simulink model "MioProgettoNew"  (R2023a)
settings: Solver=VariableStepAuto  StartTime=0.0  StopTime=10.0  RelTol=1e-3
settings Model: Creator=bened  LastModifiedBy=bened

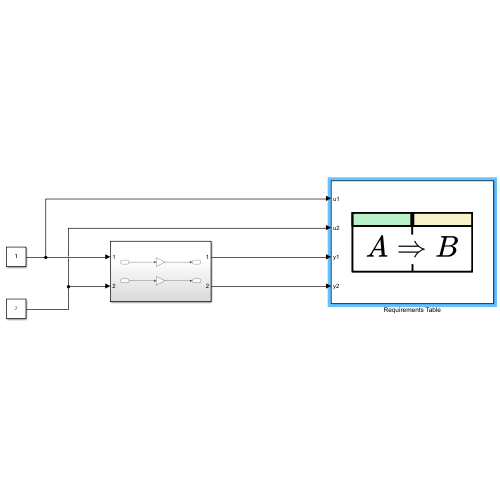
[thumbnail: Simulink's stored preview of the top-level diagram]
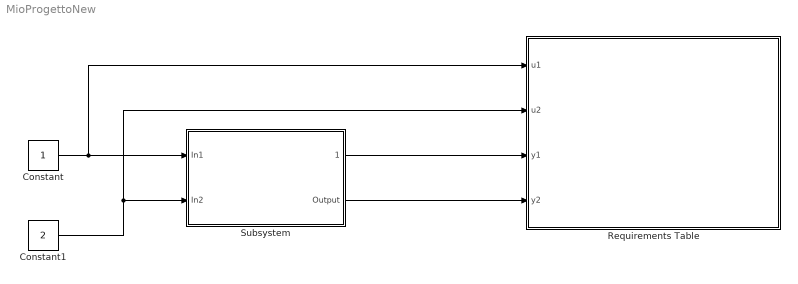
== system MioProgettoNew ==
  Constant : Constant
  Constant1 : Constant  Value=2
  Requirements Table : Requirements Table  TreatAsAtomicUnit=on
  Subsystem : Subsystem
  wires:
  Subsystem/2(Output) -> Requirements Table/4(y2)
  Subsystem/1(1) -> Requirements Table/3(y1)
  Constant/1 -> Requirements Table/1(u1), Subsystem/1(In1)
  Constant1/1 -> Subsystem/2(In2), Requirements Table/2(u2)

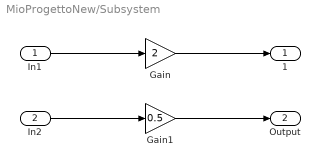
== system MioProgettoNew/Subsystem ==
  In1 : Inport
  In2 : Inport  Port=2
  Gain : Gain  Gain=2
  Gain1 : Gain  Gain=0.5
  1 : Outport
  Output : Outport  Port=2
  wires:
  In1/1 -> Gain/1
  Gain/1 -> 1/1
  In2/1 -> Gain1/1
  Gain1/1 -> Output/1

== stateflow chart MioProgettoNew/Requirements Table ==
  (default) -> (junction 1073741860)
  (junction 1073741860) -> (junction 1073741861) : {
      | % SF_REQ_REV_07
      | }
  (junction 1073741861) -> (junction 1073741863) : {
      | % HEADER_ASSIGNMENTS
      |
      | }
  (junction 1073741863) -> (junction 1073741865) : {
      | % START_A_4
      | }
  (junction 1073741865) -> (junction 1073741867) : {
      | }
  (junction 1073741867) -> (junction 1073741869)
  (junction 1073741869) -> (junction 1073741871) : {
      | }
  (junction 1073741871) -> (junction 1073741873) : {
      | % END_A_4
      | }
  (junction 1073741873) -> (junction 1073741919) : {
      | % START_R_1
      | }
  (junction 1073741919) -> (junction 1073741921) : {
      | }
  (junction 1073741921) -> (junction 1073741923)
  (junction 1073741923) -> (junction 1073741925) [order 1] : [(u1 > 0)]
  (junction 1073741923) -> (junction 1073741931) [order 2]
  (junction 1073741925) -> (junction 1073741927) : {
      | reqtable_postcondition((y1 > 0), 'R:1');
      |
      |
      | }
  (junction 1073741927) -> (junction 1073741929) : {
      | }
  (junction 1073741929) -> (junction 1073741931)
  (junction 1073741931) -> (junction 1073741933)
  (junction 1073741933) -> (junction 1073741935) : {
      | % END_R_1
      | }
  (junction 1073741935) -> (junction 1073741952) : {
      | % START_R_7
      | }
  (junction 1073741952) -> (junction 1073741954) : {
      | }
  (junction 1073741954) -> (junction 1073741956)
  (junction 1073741956) -> (junction 1073741958) [order 1] : [(u2 > 0)]
  (junction 1073741956) -> (junction 1073741964) [order 2]
  (junction 1073741958) -> (junction 1073741960) : {
      | reqtable_postcondition((y2 > 0), 'R:2');
      |
      |
      | }
  (junction 1073741960) -> (junction 1073741962) : {
      | }
  (junction 1073741962) -> (junction 1073741964)
  (junction 1073741964) -> (junction 1073741966)
  (junction 1073741966) -> (junction 1073741968) : {
      | % END_R_7
      | }
  data: u1 input; u2 input; y1 input; y2 input
